simulink model "bike_model_lqrTuning"  (R2018b)
settings: Solver=FixedStepAuto  StartTime=0.0  StopTime=sim_time  FixedStep=Ts_IMU  MaxStep=Ts  RelTol=1e-3
values from neighbouring files (symbols this model uses):
  A = [0      0            1 ... (first row only)    [lqr_design.m]
  B = [0; 1; (a_real*v*sin(lambda_real))/(h_real*b_real)]    [lqr_design.m]
  b_compFilter = 1.095    [configuration.m]    (also in configuration_lqrTuning.m)
  b_real = 1.095    [configuration.m]    (also in configuration_lqrTuning.m)
  g = 9.81    [configuration.m]    (also in configuration_lqrTuning.m)
  IMU_height_real = 0.45    [configuration.m]    (also in configuration_lqrTuning.m)
  initial_states = [deg2rad(2) deg2rad(0) deg2rad(0)]    [configuration.m]    (also in configuration_lqrTuning.m = [deg2rad(0) deg2rad(0) deg2rad(0)])
  input_velocity = 3    [configuration.m]    (also in configuration_lqrTuning.m = 4)
  lambda_compFilter = deg2rad(70)    [configuration.m]    (also in configuration_lqrTuning.m)
  lambda_real = deg2rad(70)    [configuration.m]    (also in configuration_lqrTuning.m)
  lqr_gains = zeros(length(velocity_lqr),3)    [lqr_design.m]
  parameters_compFilter = [g h_compFilter b_compFilter a_compFilter lambda_compFilter c_compFilter]    [configuration.m]    (also in configuration_lqrTuning.m)
  parameters_f_b_real = [m_frame_real m_box_real h_frame_real h_box_real a_frame_real a_box_real c_frame_real c_box_real b_frame_real b_box_real l_frame_real l_box_real]    [configuration.m]    (also in configuration_lqrTuning.m)
  parameters_real = [g h_real b_real a_real lambda_real c_real]    [configuration.m]    (also in configuration_lqrTuning.m)
  plant_model = 1    [configuration.m]    (also in configuration_lqrTuning.m = 2)
  sys_con = ss(A,B,C,D)    [lqr_design.m]
  sys_dis = c2d(sys_con,Ts)    [lqr_design.m]
  Ts = 0.04    [configuration.m]    (also in configuration_lqrTuning.m)
  Ts_IMU = 0.04    [configuration.m]    (also in configuration_lqrTuning.m)
  velocity_lqr = linspace(1.5,10,1000)    [lqr_design.m]
undefined symbols (not defined in the file or in its folder): DiscIntNeverNeededParam, initial_x, initial_y, path_x, path_y
libraries: simulink x4
settings Model: Creator=Boaz Ash  LastModifiedBy=maximef
settings DebuggingCC: UnconnectedInputMsg=none  UnconnectedOutputMsg=none  UnconnectedLineMsg=none  LibraryContextMissingDiagnostic=none
settings SFSimCC: SimUseLocalCustomCode=off
settings RTWCC: RTWUseLocalCustomCode=off

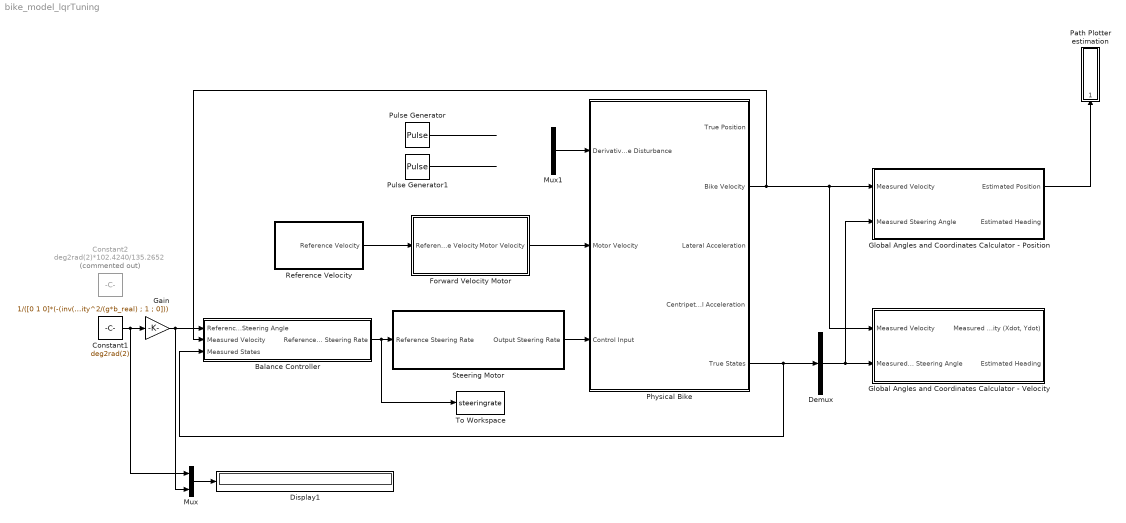
== system bike_model_lqrTuning ==
  Balance Controller : Subsystem  TreatAsAtomicUnit=on  SystemSampleTime=Ts
  Constant1 : Constant  Value=deg2rad(2)
  Constant2 : Constant  Commented=on  Value=deg2rad(2)*102.4240/135.2652
  Demux : Demux  Outputs=3
  Display1 : Display
  Forward Velocity Motor : Subsystem
  Gain : Gain  Gain=1/([0 1 0]*(-(inv(A-B*lqr_gains))*B*lqr_gains*[-input_velocity^2/(g*b_real) ; 1 ; 0]))
  Global Angles and Coordinates Calculator - Position : Subsystem  SystemSampleTime=Ts
  Global Angles and Coordinates Calculator - Velocity : Subsystem  SystemSampleTime=Ts
  Mux : Mux  Inputs=2
  Mux1 : Mux  Inputs=3
  Path Plotter estimation : Subsystem  SystemSampleTime=Ts
  Physical Bike : Subsystem
  Pulse Generator : DiscretePulseGenerator  PulseType=Time based  Amplitude=pi/36  Period=100  PhaseDelay=1
  Pulse Generator1 : DiscretePulseGenerator  PulseType=Time based  Amplitude=-deg2rad(30)  Period=10  PulseWidth=10  PhaseDelay=1
  "Reference Velocity " : Subsystem
  Steering Motor : Subsystem
  To Workspace : ToWorkspace  VariableName=steeringrate  SaveFormat=Timeseries  SampleTime=Ts
  wires:
  Pulse Generator/1 -> ?
  Pulse Generator1/1 -> ?
  Physical Bike/2(Bike Velocity) -> Balance Controller/2(Measured Velocity), Global Angles and Coordinates Calculator - Velocity/1(Measured Velocity), Global Angles and Coordinates Calculator - Position/1(Measured Velocity)
  Forward Velocity Motor/1(Motor Velocity) -> Physical Bike/2(Motor Velocity)
  "Reference Velocity "/1(Reference Velocity) -> Forward Velocity Motor/1(Reference Velocity)
  Steering Motor/1(Output Steering Rate) -> Physical Bike/3(Control Input)
  Physical Bike/5(True States) -> Balance Controller/3(Measured States), Demux/1
  Demux/2 -> Global Angles and Coordinates Calculator - Velocity/2("Measured Steering Angle "), Global Angles and Coordinates Calculator - Position/2(Measured Steering Angle)
  Mux1/1 -> Physical Bike/1(Derivative Disturbance)
  Global Angles and Coordinates Calculator - Position/1(Estimated Position) -> Path Plotter estimation/1(Position)
  Balance Controller/1(Reference Steering Rate) -> To Workspace/1, Steering Motor/1(Reference Steering Rate)
  Constant1/1 -> Mux/1, Gain/1
  Gain/1 -> Mux/2, Balance Controller/1(Reference Steering Angle)
  Mux/1 -> Display1/1

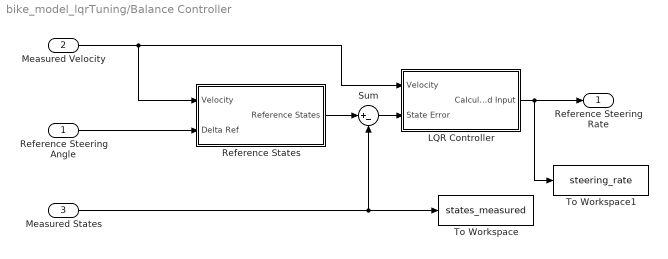
== system bike_model_lqrTuning/Balance Controller ==
  Reference Steering Angle : Inport
  Measured Velocity : Inport  Port=2
  Measured States : Inport  Port=3
  LQR Controller : Subsystem  TreatAsAtomicUnit=on  SystemSampleTime=Ts
  Reference States : Subsystem  SystemSampleTime=Ts
  Sum : Sum  Inputs=|+-
  To Workspace : ToWorkspace  VariableName=states_measured  SaveFormat=Timeseries  SampleTime=-1
  To Workspace1 : ToWorkspace  VariableName=steering_rate  SaveFormat=Timeseries  SampleTime=-1
  Reference Steering Rate : Outport
  wires:
  Reference States/1(Reference States) -> Sum/1
  Sum/1 -> LQR Controller/2(State Error)
  LQR Controller/1(Calculated Input) -> To Workspace1/1, Reference Steering Rate/1
  Reference Steering Angle/1 -> Reference States/2(Delta Ref)
  Measured Velocity/1 -> Reference States/1(Velocity), LQR Controller/1(Velocity)
  Measured States/1 -> To Workspace/1, Sum/2

== system bike_model_lqrTuning/Forward Velocity Motor ==
  note: Add limit for acceleration/deceleration
      | Add min speed of 1.69 m/s (3600 rpm motor speed) limitation
      | Add min speed of 8.20 m/s (18000 rpm motor speed) limitation
      | Add deadband and delay
  Reference Velocity : Inport
  Motor Velocity : Outport
  wires:
  Reference Velocity/1 -> Motor Velocity/1

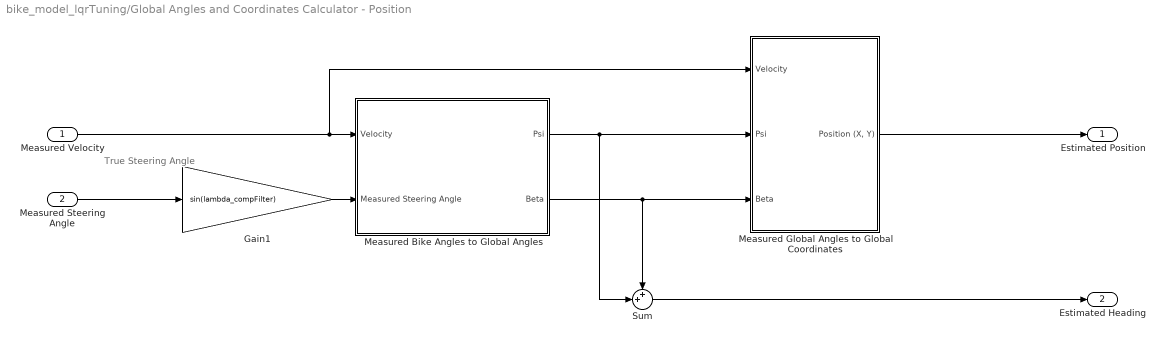
== system bike_model_lqrTuning/Global Angles and Coordinates Calculator - Position ==
  note: True Steering
      | Angle
  Measured Velocity : Inport
  Measured Steering Angle : Inport  Port=2
  Gain1 : Gain  Gain=sin(lambda_compFilter)
  Measured Bike Angles to Global Angles : Subsystem
  Measured Global Angles to Global Coordinates : Subsystem
  Sum : Sum  Inputs=++|
  Estimated Position : Outport
  Estimated Heading : Outport  Port=2
  wires:
  Measured Bike Angles to Global Angles/1(Psi) -> Sum/2, Measured Global Angles to Global Coordinates/2(Psi)
  Gain1/1 -> Measured Bike Angles to Global Angles/2(Measured Steering Angle)
  Sum/1 -> Estimated Heading/1
  Measured Bike Angles to Global Angles/2(Beta) -> Sum/1, Measured Global Angles to Global Coordinates/3(Beta)
  Measured Global Angles to Global Coordinates/1("Position (X, Y)") -> Estimated Position/1
  Measured Velocity/1 -> Measured Global Angles to Global Coordinates/1(Velocity), Measured Bike Angles to Global Angles/1(Velocity)
  Measured Steering Angle/1 -> Gain1/1

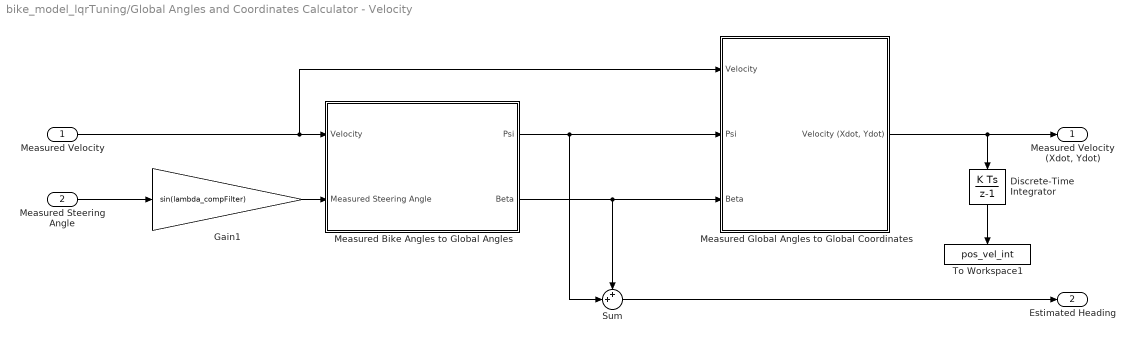
== system bike_model_lqrTuning/Global Angles and Coordinates Calculator - Velocity ==
  Measured Velocity : Inport
  "Measured Steering Angle " : Inport  Port=2
  Discrete-Time Integrator : DiscreteIntegrator  SampleTime=-1  ICPrevOutput=DiscIntNeverNeededParam  ICPrevScaledInput=DiscIntNeverNeededParam
  Gain1 : Gain  Gain=sin(lambda_compFilter)
  Measured Bike Angles to Global Angles : Subsystem
  Measured Global Angles to Global Coordinates : Subsystem
  Sum : Sum  Inputs=++|
  To Workspace1 : ToWorkspace  VariableName=pos_vel_int  SaveFormat=Timeseries  SampleTime=-1
  "Measured Velocity (Xdot, Ydot)" : Outport
  Estimated Heading : Outport  Port=2
  wires:
  "Measured Steering Angle "/1 -> Gain1/1
  Measured Bike Angles to Global Angles/1(Psi) -> Sum/2, Measured Global Angles to Global Coordinates/2(Psi)
  Gain1/1 -> Measured Bike Angles to Global Angles/2(Measured Steering Angle)
  Sum/1 -> Estimated Heading/1
  Measured Bike Angles to Global Angles/2(Beta) -> Measured Global Angles to Global Coordinates/3(Beta), Sum/1
  Measured Velocity/1 -> Measured Bike Angles to Global Angles/1(Velocity), Measured Global Angles to Global Coordinates/1(Velocity)
  Measured Global Angles to Global Coordinates/1("Velocity (Xdot, Ydot)") -> "Measured Velocity (Xdot, Ydot)"/1, Discrete-Time Integrator/1
  Discrete-Time Integrator/1 -> To Workspace1/1

== system bike_model_lqrTuning/Path Plotter estimation ==
  Position : Inport
  Demux : Demux  Outputs=2
  To Workspace : ToWorkspace  VariableName=X_BIKE_estim  SaveFormat=Timeseries  SampleTime=Ts
  To Workspace1 : ToWorkspace  VariableName=Y_BIKE_estim  SaveFormat=Timeseries  SampleTime=Ts
  XY Graph : simulink/Sinks/XY Graph  Commented=on  xmin=min(path_x)-5  xmax=max(path_x)+5  ymin=min(path_y)-5  ymax=max(path_y)+5  st=-1
  wires:
  Demux/1 -> XY Graph/1, To Workspace/1  "X"
  Demux/2 -> XY Graph/2, To Workspace1/1  "Y"
  Position/1 -> Demux/1

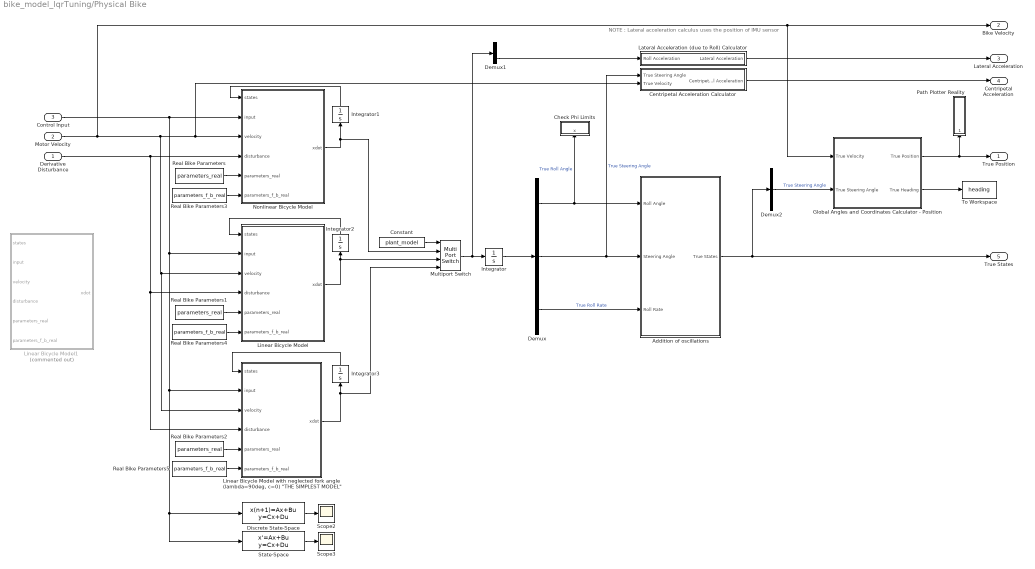
== system bike_model_lqrTuning/Physical Bike ==
  note: NOTE : Lateral acceleration calculus uses the position of IMU sensor
  Derivative Disturbance : Inport
  Motor Velocity : Inport  Port=2
  Control Input : Inport  Port=3
  " Addition of oscillations" : Subsystem  SystemSampleTime=Ts
  Centripetal Acceleration Calculator : Subsystem
  Check Phi Limits : Subsystem  TreatAsAtomicUnit=on  SystemSampleTime=Ts
  Constant : Constant  Value=plant_model
  Demux : Demux  Outputs=3
  Demux1 : Demux  Outputs=3
  Demux2 : Demux  Outputs=3
  Discrete State-Space : DiscreteStateSpace  A=sys_dis.A  B=sys_dis.B  C=eye(3,3)  D=zeros(3,1)  SampleTime=Ts_IMU
  Global Angles and Coordinates Calculator - Position : Subsystem  SystemSampleTime=Ts
  Integrator{,1..3} (4 alike) : Integrator  InitialCondition=initial_states
  Lateral Acceleration (due to Roll) Calculator : Subsystem
  Linear Bicycle Model : MATLAB Function  TreatAsAtomicUnit=on
  "Linear Bicycle Model with neglected fork angle (lambda=90deg, c=0) \"THE SIMPLEST MODEL\"" : MATLAB Function  TreatAsAtomicUnit=on
  Linear Bicycle Model1 : MATLAB Function  Commented=on  TreatAsAtomicUnit=on
  Multiport Switch : MultiPortSwitch
  Nonlinear Bicycle Model : MATLAB Function  TreatAsAtomicUnit=on
  Path Plotter Reality : Subsystem  SystemSampleTime=Ts
  Real Bike Parameters : Constant  Value=parameters_real
  Real Bike Parameters1 : Constant  Value=parameters_real
  Real Bike Parameters2 : Constant  Value=parameters_real
  Real Bike Parameters3 : Constant  Value=parameters_f_b_real
  Real Bike Parameters4 : Constant  Value=parameters_f_b_real
  Real Bike Parameters5 : Constant  Value=parameters_f_b_real
  Scope2 : Scope
  Scope3 : Scope
  State-Space : StateSpace  A=sys_con.A  B=sys_con.B  C=eye(3,3)  D=zeros(3,1)  InitialCondition=0
  To Workspace : ToWorkspace  VariableName=heading  SaveFormat=Timeseries  SampleTime=Ts
  True Position : Outport
  Bike Velocity : Outport  Port=2
  Lateral Acceleration : Outport  Port=3
  Centripetal Acceleration : Outport  Port=4
  True States : Outport  Port=5
  wires:
  Real Bike Parameters5/1 -> "Linear Bicycle Model with neglected fork angle (lambda=90deg, c=0) \"THE SIMPLEST MODEL\""/6(parameters_f_b_real)
  Demux/2 -> Centripetal Acceleration Calculator/1(True Steering Angle), " Addition of oscillations"/2(Steering Angle)  "True Steering Angle"
  Control Input/1 -> Nonlinear Bicycle Model/2(input), State-Space/1, Discrete State-Space/1, "Linear Bicycle Model with neglected fork angle (lambda=90deg, c=0) \"THE SIMPLEST MODEL\""/2(input), Linear Bicycle Model/2(input)
  Integrator1/1 -> Nonlinear Bicycle Model/1(states)
  Real Bike Parameters3/1 -> Nonlinear Bicycle Model/6(parameters_f_b_real)
  Constant/1 -> Multiport Switch/1
  Real Bike Parameters2/1 -> "Linear Bicycle Model with neglected fork angle (lambda=90deg, c=0) \"THE SIMPLEST MODEL\""/5(parameters_real)
  State-Space/1 -> Scope3/1
  Discrete State-Space/1 -> Scope2/1
  Integrator/1 -> Demux/1
  Demux/1 -> Check Phi Limits/1(x), " Addition of oscillations"/1(Roll Angle)  "True Roll Angle"
  Real Bike Parameters1/1 -> Linear Bicycle Model/5(parameters_real)
  Centripetal Acceleration Calculator/1(Centripetal Acceleration) -> Centripetal Acceleration/1
  Nonlinear Bicycle Model/1(xdot) -> Integrator1/1, Multiport Switch/2
  Demux1/3 -> Lateral Acceleration (due to Roll) Calculator/1(Roll Acceleration)
  Linear Bicycle Model/1(xdot) -> Integrator2/1, Multiport Switch/3
  Derivative Disturbance/1 -> Nonlinear Bicycle Model/4(disturbance), "Linear Bicycle Model with neglected fork angle (lambda=90deg, c=0) \"THE SIMPLEST MODEL\""/4(disturbance), Linear Bicycle Model/4(disturbance)
  Real Bike Parameters/1 -> Nonlinear Bicycle Model/5(parameters_real)
  "Linear Bicycle Model with neglected fork angle (lambda=90deg, c=0) \"THE SIMPLEST MODEL\""/1(xdot) -> Integrator3/1, Multiport Switch/4
  Multiport Switch/1 -> Demux1/1, Integrator/1
  Lateral Acceleration (due to Roll) Calculator/1(Lateral Acceleration) -> Lateral Acceleration/1
  Integrator3/1 -> "Linear Bicycle Model with neglected fork angle (lambda=90deg, c=0) \"THE SIMPLEST MODEL\""/1(states)
  Integrator2/1 -> Linear Bicycle Model/1(states)
  Motor Velocity/1 -> Global Angles and Coordinates Calculator - Position/1(True Velocity), Bike Velocity/1, Nonlinear Bicycle Model/3(velocity), Centripetal Acceleration Calculator/2(True Velocity), "Linear Bicycle Model with neglected fork angle (lambda=90deg, c=0) \"THE SIMPLEST MODEL\""/3(velocity), Linear Bicycle Model/3(velocity)
  Real Bike Parameters4/1 -> Linear Bicycle Model/6(parameters_f_b_real)
  Demux/3 -> " Addition of oscillations"/3(Roll Rate)  "True Roll Rate"
  " Addition of oscillations"/1(True States) -> Demux2/1, True States/1
  Demux2/2 -> Global Angles and Coordinates Calculator - Position/2(True Steering Angle)  "True Steering Angle"
  Global Angles and Coordinates Calculator - Position/1(True Position) -> True Position/1, Path Plotter Reality/1(Position)
  Global Angles and Coordinates Calculator - Position/2(True Heading) -> To Workspace/1

== system bike_model_lqrTuning/Reference Velocity  ==
  Constant Velocity : Constant  Value=input_velocity
  Reference Velocity : Outport
  wires:
  Constant Velocity/1 -> Reference Velocity/1

== system bike_model_lqrTuning/Steering Motor ==
  Reference Steering Rate : Inport
  To Workspace : ToWorkspace  VariableName=calculated_input  SaveFormat=Timeseries  SampleTime=Ts
  To Workspace1 : ToWorkspace  VariableName=realised_input  SaveFormat=Timeseries  SampleTime=Ts
  Output Steering Rate : Outport
  wires:
  Reference Steering Rate/1 -> Output Steering Rate/1, To Workspace1/1, To Workspace/1

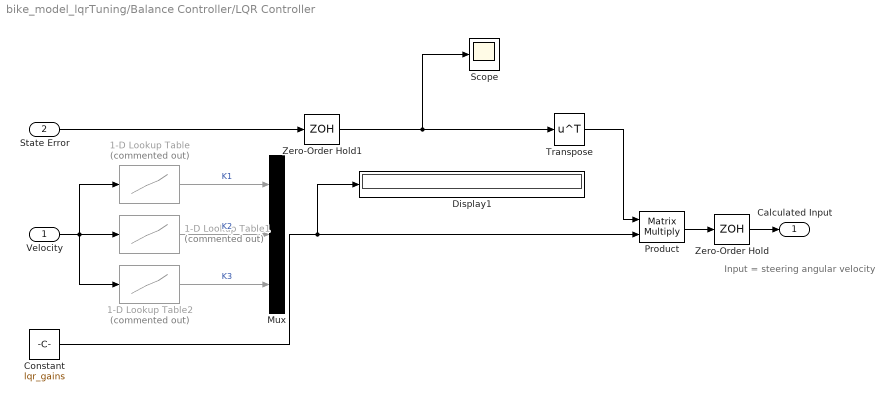
== system bike_model_lqrTuning/Balance Controller/LQR Controller ==
  note: Input = steering angular velocity
  Velocity : Inport
  State Error : Inport  Port=2
  1-D Lookup Table : Lookup_n-D  Commented=on  NumberOfTableDimensions=1  BreakpointsForDimension1=velocity_lqr  BreakpointsForDimension2=velocity_lqr  BreakpointsForDimension3=velocity_lqr  BreakpointsForDimension4=velocity_lqr  Table=lqr_gains(:,1)  InternalRulePriority=Speed  RndMeth=Simplest  InputSameDT=on
  1-D Lookup Table1 : Lookup_n-D  Commented=on  NumberOfTableDimensions=1  BreakpointsForDimension1=velocity_lqr  BreakpointsForDimension2=velocity_lqr  BreakpointsForDimension3=velocity_lqr  BreakpointsForDimension4=velocity_lqr  Table=lqr_gains(:,2)  InternalRulePriority=Speed  RndMeth=Simplest  InputSameDT=on
  1-D Lookup Table2 : Lookup_n-D  Commented=on  NumberOfTableDimensions=1  BreakpointsForDimension1=velocity_lqr  BreakpointsForDimension2=velocity_lqr  BreakpointsForDimension3=velocity_lqr  BreakpointsForDimension4=velocity_lqr  Table=lqr_gains(:,3)  InternalRulePriority=Speed  RndMeth=Simplest  InputSameDT=on
  Constant : Constant  Value=lqr_gains
  Display1 : Display
  Mux : Mux  Inputs=3
  Product : Product  Multiplication=Matrix(*)
  Scope : Scope
  Transpose : Math  Operator=transpose  SaturateOnIntegerOverflow=on
  Zero-Order Hold : ZeroOrderHold  SampleTime=Ts
  Zero-Order Hold1 : ZeroOrderHold  SampleTime=Ts
  Calculated Input : Outport
  wires:
  1-D Lookup Table/1 -> Mux/1  "K1"
  1-D Lookup Table1/1 -> Mux/2  "K2"
  State Error/1 -> Zero-Order Hold1/1
  Product/1 -> Zero-Order Hold/1
  1-D Lookup Table2/1 -> Mux/3  "K3"
  Velocity/1 -> 1-D Lookup Table2/1, 1-D Lookup Table1/1, 1-D Lookup Table/1
  Constant/1 -> Product/2, Display1/1
  Transpose/1 -> Product/1
  Zero-Order Hold/1 -> Calculated Input/1
  Zero-Order Hold1/1 -> Scope/1, Transpose/1

== system bike_model_lqrTuning/Balance Controller/Reference States ==
  Velocity : Inport
  Delta Ref : Inport  Port=2
  Bike Parameters : Constant  Value=parameters_real
  Mux5 : Mux  Inputs=3
  Reference Roll Angle Calculator : MATLAB Function  Commented=on  TreatAsAtomicUnit=on
  Reference Roll Angle Calculator_lin : MATLAB Function  TreatAsAtomicUnit=on
  Reference States : Outport
  wires:
  Bike Parameters/1 -> Reference Roll Angle Calculator_lin/1(parameters_real)
  Delta Ref/1 -> Mux5/2, Reference Roll Angle Calculator_lin/3(delta_ref)
  Reference Roll Angle Calculator_lin/1(phi_ref) -> Mux5/1
  Velocity/1 -> Reference Roll Angle Calculator_lin/2(velocity)
  Mux5/1 -> Reference States/1

== system bike_model_lqrTuning/Global Angles and Coordinates Calculator - Position/Measured Bike Angles to Global Angles ==
  Velocity : Inport
  Measured Steering Angle : Inport  Port=2
  " Bike Parameters Model " : Constant  Value=parameters_compFilter
  Integrator : Integrator
  MATLAB Function : MATLAB Function  TreatAsAtomicUnit=on
  Psi : Outport
  Beta : Outport  Port=2
  wires:
  MATLAB Function/2(beta) -> Beta/1
  MATLAB Function/1(psi_d) -> Integrator/1
  Integrator/1 -> Psi/1
  " Bike Parameters Model "/1 -> MATLAB Function/2(parameters_model)
  Measured Steering Angle/1 -> MATLAB Function/3(delta)
  Velocity/1 -> MATLAB Function/1(v)

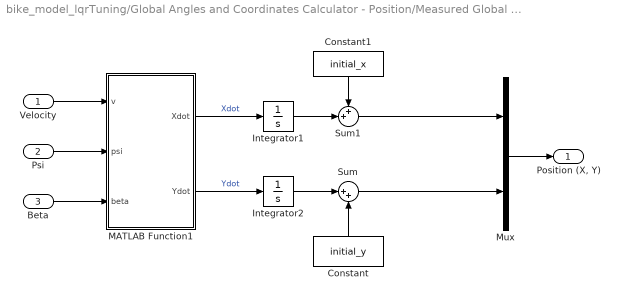
== system bike_model_lqrTuning/Global Angles and Coordinates Calculator - Position/Measured Global Angles to Global Coordinates ==
  Velocity : Inport
  Psi : Inport  Port=2
  Beta : Inport  Port=3
  Constant : Constant  Value=initial_y
  Constant1 : Constant  Value=initial_x
  Integrator1 : Integrator
  Integrator2 : Integrator
  MATLAB Function1 : MATLAB Function  TreatAsAtomicUnit=on
  Mux : Mux  Inputs=2
  Sum : Sum  Inputs=|++
  Sum1 : Sum  Inputs=++|
  "Position (X, Y)" : Outport
  wires:
  MATLAB Function1/2(Ydot) -> Integrator2/1  "Ydot"
  MATLAB Function1/1(Xdot) -> Integrator1/1  "Xdot"
  Psi/1 -> MATLAB Function1/2(psi)
  Beta/1 -> MATLAB Function1/3(beta)
  Velocity/1 -> MATLAB Function1/1(v)
  Integrator2/1 -> Sum/1
  Constant/1 -> Sum/2
  Sum/1 -> Mux/2
  Integrator1/1 -> Sum1/2
  Sum1/1 -> Mux/1
  Constant1/1 -> Sum1/1
  Mux/1 -> "Position (X, Y)"/1

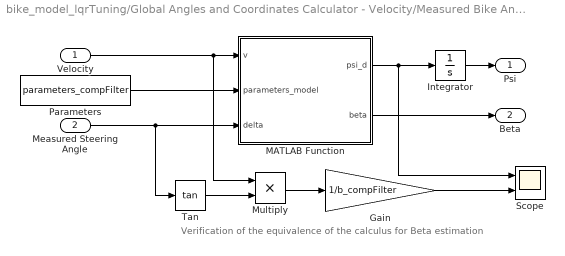
== system bike_model_lqrTuning/Global Angles and Coordinates Calculator - Velocity/Measured Bike Angles to Global Angles ==
  note: Verification of the equivalence of the calculus for Beta estimation
  Velocity : Inport
  Measured Steering Angle : Inport  Port=2
  Gain : Gain  Gain=1/b_compFilter
  Integrator : Integrator
  MATLAB Function : MATLAB Function  TreatAsAtomicUnit=on
  Multiply : Product
  Parameters : Constant  Value=parameters_compFilter
  Scope : Scope  NumInputPorts=2
  Tan : Trigonometry  Operator=tan
  Psi : Outport
  Beta : Outport  Port=2
  wires:
  Integrator/1 -> Psi/1
  MATLAB Function/1(psi_d) -> Scope/1, Integrator/1
  Measured Steering Angle/1 -> Tan/1, MATLAB Function/3(delta)
  Parameters/1 -> MATLAB Function/2(parameters_model)
  Velocity/1 -> Multiply/1, MATLAB Function/1(v)
  MATLAB Function/2(beta) -> Beta/1
  Tan/1 -> Multiply/2
  Multiply/1 -> Gain/1
  Gain/1 -> Scope/2

== system bike_model_lqrTuning/Global Angles and Coordinates Calculator - Velocity/Measured Global Angles to Global Coordinates ==
  Velocity : Inport
  Psi : Inport  Port=2
  Beta : Inport  Port=3
  MATLAB Function1 : MATLAB Function  TreatAsAtomicUnit=on
  Mux1 : Mux  Inputs=2
  "Velocity (Xdot, Ydot)" : Outport
  wires:
  MATLAB Function1/2(Ydot) -> Mux1/2  "Ydot"
  MATLAB Function1/1(Xdot) -> Mux1/1  "Xdot"
  Psi/1 -> MATLAB Function1/2(psi)
  Beta/1 -> MATLAB Function1/3(beta)
  Velocity/1 -> MATLAB Function1/1(v)
  Mux1/1 -> "Velocity (Xdot, Ydot)"/1

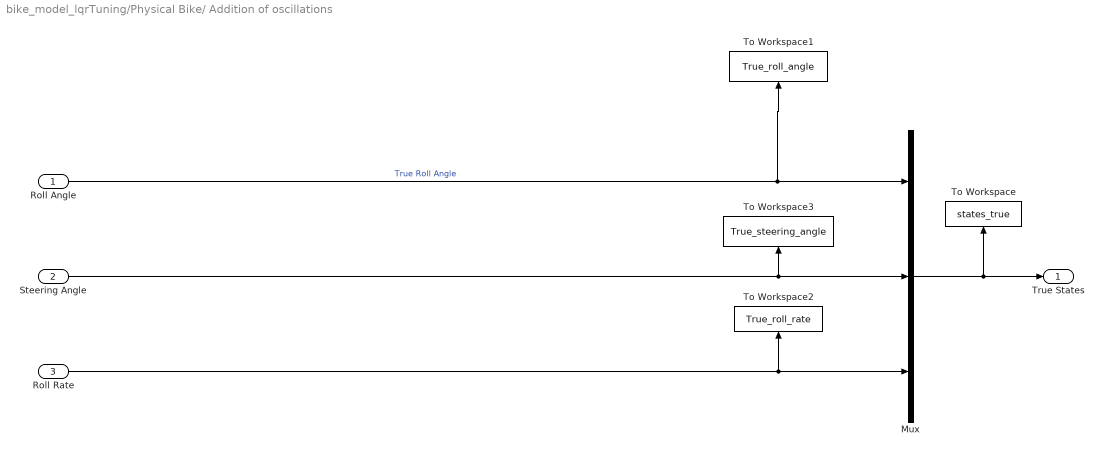
== system bike_model_lqrTuning/Physical Bike/ Addition of oscillations ==
  Roll Angle : Inport
  Steering Angle : Inport  Port=2
  Roll Rate : Inport  Port=3
  Mux : Mux  Inputs=3
  To Workspace : ToWorkspace  VariableName=states_true  SaveFormat=Timeseries  SampleTime=Ts
  To Workspace1 : ToWorkspace  VariableName=True_roll_angle  SaveFormat=Structure  SampleTime=Ts
  To Workspace2 : ToWorkspace  VariableName=True_roll_rate  SaveFormat=Structure  SampleTime=Ts
  To Workspace3 : ToWorkspace  VariableName=True_steering_angle  SaveFormat=Structure  SampleTime=-1
  True States : Outport
  wires:
  Steering Angle/1 -> To Workspace3/1, Mux/2
  Roll Rate/1 -> Mux/3, To Workspace2/1
  Roll Angle/1 -> To Workspace1/1, Mux/1  "True Roll Angle"
  Mux/1 -> True States/1, To Workspace/1

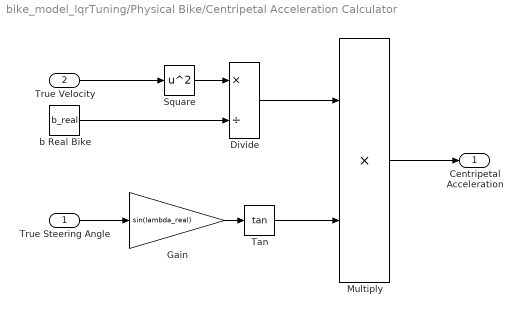
== system bike_model_lqrTuning/Physical Bike/Centripetal Acceleration Calculator ==
  True Steering Angle : Inport
  True Velocity : Inport  Port=2
  Divide : Product  Inputs=*/
  Gain : Gain  Gain=sin(lambda_real)
  Multiply : Product
  Square : Math  Operator=square  SaturateOnIntegerOverflow=on
  Tan : Trigonometry  Operator=tan
  b Real Bike : Constant  Value=b_real
  Centripetal Acceleration : Outport
  wires:
  True Velocity/1 -> Square/1
  Square/1 -> Divide/1
  b Real Bike/1 -> Divide/2
  True Steering Angle/1 -> Gain/1
  Divide/1 -> Multiply/1
  Tan/1 -> Multiply/2
  Multiply/1 -> Centripetal Acceleration/1
  Gain/1 -> Tan/1

== system bike_model_lqrTuning/Physical Bike/Check Phi Limits ==
  x : Inport
  Roll Lower Bound : simulink/Model Verification/Check Static  Lower Bound  Description=min_roll <= u  min=min_roll  min_included=on  enabled=on  stopWhenAssertionFail=on  export=off  icon=graphic
      settings: SourceProductName=Simulink
  Roll Upper Bound : simulink/Model Verification/Check Static  Upper Bound  Description=u <= max_roll  max=max_roll  max_included=on  enabled=on  stopWhenAssertionFail=on  export=off  icon=graphic
      settings: SourceProductName=Simulink  SourceProductBaseCode=SL
  wires:
  x/1 -> Roll Lower Bound/1, Roll Upper Bound/1  "Roll Angle"

== system bike_model_lqrTuning/Physical Bike/Global Angles and Coordinates Calculator - Position ==
  note: True Steering
      | Angle
  True Velocity : Inport
  True Steering Angle : Inport  Port=2
  Gain1 : Gain  Gain=sin(lambda_compFilter)
  Measured Bike Angles to Global Angles : Subsystem
  Measured Global Angles to Global Coordinates : Subsystem
  Sum : Sum  Inputs=++|
  True Position : Outport
  True Heading : Outport  Port=2
  wires:
  Measured Bike Angles to Global Angles/1(Psi) -> Sum/2, Measured Global Angles to Global Coordinates/2(Psi)
  Gain1/1 -> Measured Bike Angles to Global Angles/2(Measured Steering Angle)
  Sum/1 -> True Heading/1
  Measured Bike Angles to Global Angles/2(Beta) -> Sum/1, Measured Global Angles to Global Coordinates/3(Beta)
  Measured Global Angles to Global Coordinates/1("Position (X, Y)") -> True Position/1
  True Velocity/1 -> Measured Global Angles to Global Coordinates/1(Velocity), Measured Bike Angles to Global Angles/1(Velocity)
  True Steering Angle/1 -> Gain1/1

== system bike_model_lqrTuning/Physical Bike/Lateral Acceleration (due to Roll) Calculator ==
  Roll Acceleration : Inport
  Constant3 : Constant  Value=IMU_height_real
  Multiply : Product
  Lateral Acceleration : Outport
  wires:
  Multiply/1 -> Lateral Acceleration/1
  Constant3/1 -> Multiply/1
  Roll Acceleration/1 -> Multiply/2

== system bike_model_lqrTuning/Physical Bike/Path Plotter Reality ==
  Position : Inport
  Demux : Demux  Outputs=2
  To Workspace : ToWorkspace  VariableName=X_BIKE  SaveFormat=Timeseries  SampleTime=Ts
  To Workspace1 : ToWorkspace  VariableName=Y_BIKE  SaveFormat=Timeseries  SampleTime=Ts
  XY Graph : simulink/Sinks/XY Graph  Commented=on  xmin=min(path_x)-5  xmax=max(path_x)+5  ymin=min(path_y)-5  ymax=max(path_y)+5  st=-1
  wires:
  Demux/1 -> XY Graph/1, To Workspace/1  "X"
  Demux/2 -> XY Graph/2, To Workspace1/1  "Y"
  Position/1 -> Demux/1

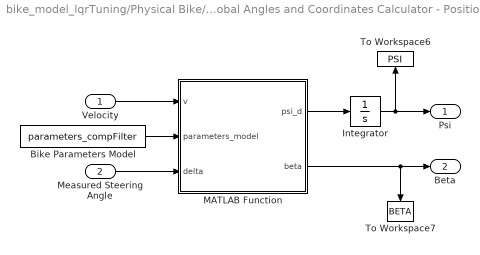
== system bike_model_lqrTuning/Physical Bike/Global Angles and Coordinates Calculator - Position/Measured Bike Angles to Global Angles ==
  Velocity : Inport
  Measured Steering Angle : Inport  Port=2
  " Bike Parameters Model " : Constant  Value=parameters_compFilter
  Integrator : Integrator
  MATLAB Function : MATLAB Function  TreatAsAtomicUnit=on
  To Workspace6 : ToWorkspace  VariableName=PSI  SaveFormat=Timeseries  SampleTime=Ts
  To Workspace7 : ToWorkspace  VariableName=BETA  SaveFormat=Timeseries  SampleTime=Ts
  Psi : Outport
  Beta : Outport  Port=2
  wires:
  MATLAB Function/2(beta) -> Beta/1, To Workspace7/1
  MATLAB Function/1(psi_d) -> Integrator/1
  Integrator/1 -> Psi/1, To Workspace6/1
  " Bike Parameters Model "/1 -> MATLAB Function/2(parameters_model)
  Measured Steering Angle/1 -> MATLAB Function/3(delta)
  Velocity/1 -> MATLAB Function/1(v)

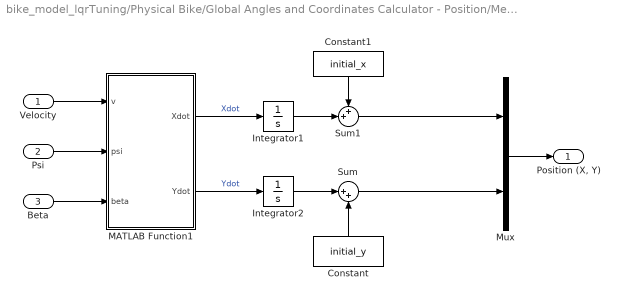
== system bike_model_lqrTuning/Physical Bike/Global Angles and Coordinates Calculator - Position/Measured Global Angles to Global Coordinates ==
  Velocity : Inport
  Psi : Inport  Port=2
  Beta : Inport  Port=3
  Constant : Constant  Value=initial_y
  Constant1 : Constant  Value=initial_x
  Integrator1 : Integrator
  Integrator2 : Integrator
  MATLAB Function1 : MATLAB Function  TreatAsAtomicUnit=on
  Mux : Mux  Inputs=2
  Sum : Sum  Inputs=|++
  Sum1 : Sum  Inputs=++|
  "Position (X, Y)" : Outport
  wires:
  MATLAB Function1/2(Ydot) -> Integrator2/1  "Ydot"
  MATLAB Function1/1(Xdot) -> Integrator1/1  "Xdot"
  Psi/1 -> MATLAB Function1/2(psi)
  Beta/1 -> MATLAB Function1/3(beta)
  Velocity/1 -> MATLAB Function1/1(v)
  Integrator2/1 -> Sum/1
  Constant/1 -> Sum/2
  Sum/1 -> Mux/2
  Integrator1/1 -> Sum1/2
  Sum1/1 -> Mux/1
  Constant1/1 -> Sum1/1
  Mux/1 -> "Position (X, Y)"/1

== matlab function bike_model_lqrTuning/Balance Controller/Reference States/Reference Roll Angle Calculator_lin ==
  data: parameters_real input; velocity input; delta_ref input; phi_ref output
function phi_ref = fcn(parameters_real, velocity, delta_ref)
g = parameters_real(1);
b = parameters_real(3);
v = velocity;

phi_ref = -(v^2 / (g * b) * delta_ref); % tan(theta_ref));

== matlab function bike_model_lqrTuning/Physical Bike/Linear Bicycle Model ==
  data: states input; input input; xdot output; velocity input; disturbance input; parameters_real input; parameters_f_b_real input
function xdot = fcn(states,input,velocity,disturbance,parameters_real,parameters_f_b_real)

delta_d=input;
v=velocity;
d1=disturbance(1);
d2=disturbance(2);
d3=disturbance(3);

% % % 1=frame | 2=box
% % m1=parameters_f_b_real(1);
% % m2=parameters_f_b_real(2);
% % h1=parameters_f_b_real(3);
% % h2=parameters_f_b_real(4);
% % a1=parameters_f_b_real(5);
% % a2=parameters_f_b_real(6);
% % c1=parameters_f_b_real(7);
% % c2=parameters_f_b_real(8);
% % b1=parameters_f_b_real(9);
% % b2=parameters_f_b_real(10);
% % l1=parameters_f_b_real(11);
% % l2=parameters_f_b_real(12);

% 1=frame | 2=box
m1=parameters_real(1);
m2=parameters_real(1);
h1=parameters_real(2);
h2=parameters_real(2);
a1=parameters_real(3);
a2=parameters_real(3);
c1=parameters_real(4);
c2=parameters_real(4);
b1=parameters_real(5);
b2=parameters_real(5);
l1=parameters_real(6);
l2=parameters_real(6);

g=parameters_real(1);
h=parameters_real(2);
b=parameters_real(3);
a=parameters_real(4);
lambda=parameters_real(5);
c=parameters_real(6);

phi=states(1);
delta=states(2);
phi_d=states(3);

A=((m1/12)*((c1^2)+(b1^2)))+(m1*(h1^2))+((m2/12)*((c2^2)+(b2^2)))+(m2*(h2^2));
B=((m1/12)*((l1^2)+(b1^2)))-(m1*a1*h1)+((m2/12)*((c2^2)+(b2^2)))+(m2*a2*h2);
D=(((m1*h1)+(m2*h2))*(v^2))-(c*g*((m1*a1)-(m2*a2)));

xdot1=phi_d+d1;
xdot2=delta_d+d2;
% xdot3=((((m1*h1)+(m2*h2))*g)/A)*phi+((D*sin(lambda))/(b*A))*delta+d3+((B*v*sin(lambda))/(b*A))*delta_d;
xdot3=(g/h)*phi+(sin(lambda)*(h*v^2-g*a*c)/(h^2*b))*delta+d3+((a*v*sin(lambda))/(h*b))*delta_d;

xdot=[xdot1 xdot2 xdot3];

== matlab function bike_model_lqrTuning/Global Angles and Coordinates Calculator - Position/Measured Bike Angles to Global Angles/MATLAB Function ==
  data: v input; parameters_model input; delta input; psi_d output; beta output
function [psi_d, beta]  = fcn(v, parameters_model, delta)

b = parameters_model(3);
a = parameters_model(4);

beta = atan((a / (b)) * tan(delta));
psi_d = (v / a) * sin(beta);

== matlab function bike_model_lqrTuning/Physical Bike/Linear Bicycle Model1 ==
  data: states input; input input; xdot output; velocity input; disturbance input; parameters_real input; parameters_f_b_real input
function xdot = fcn(states,input,velocity,disturbance,parameters_real,parameters_f_b_real)

delta_d=input;
v=velocity;
d1=disturbance(1);
d2=disturbance(2);
d3=disturbance(3);

% 1=frame | 2=box
m1=parameters_f_b_real(1);
m2=parameters_f_b_real(2);
h1=parameters_f_b_real(3);
h2=parameters_f_b_real(4);
a1=parameters_f_b_real(5);
a2=parameters_f_b_real(6);
c1=parameters_f_b_real(7);
c2=parameters_f_b_real(8);
b1=parameters_f_b_real(9);
b2=parameters_f_b_real(10);
l1=parameters_f_b_real(11);
l2=parameters_f_b_real(12);

g=parameters_real(1);
%h=parameters_real(2);
b=parameters_real(3);
%a=parameters_real(4);
lambda=parameters_real(5);
c=parameters_real(6);

phi=states(1);
delta=states(2);
phi_d=states(3);

A=((m1/12)*((c1^2)+(b1^2)))+(m1*(h1^2))+((m2/12)*((c2^2)+(b2^2)))+(m2*(h2^2));
B=((m1/12)*((l1^2)+(b1^2)))-(m1*a1*h1)+((m2/12)*((c2^2)+(b2^2)))+(m2*a2*h2);
D=(((m1*h1)+(m2*h2))*(v^2))-(c*g*((m1*a1)-(m2*a2)));

xdot1=phi_d+d1;
xdot2=delta_d+d2;
xdot3=((((m1*h1)+(m2*h2))*g)/A)*phi+((D*sin(lambda))/(b*A))*delta+d3+((B*v*sin(lambda))/(b*A))*delta_d;

xdot=[xdot1 xdot2 xdot3];

== matlab function bike_model_lqrTuning/Global Angles and Coordinates Calculator - Position/Measured Global Angles to Global Coordinates/MATLAB Function1 ==
  data: v input; psi input; Xdot output; beta input; Ydot output
function [Xdot, Ydot]  = fcn(v, psi, beta)

Xdot = v * cos(psi + beta);
Ydot = v * sin(psi + beta);

== matlab function bike_model_lqrTuning/Balance Controller/Reference States/Reference Roll Angle Calculator ==
  data: parameters_real input; velocity input; delta_ref input; phi_ref output
function phi_ref = fcn(parameters_real, velocity, delta_ref)
g = parameters_real(1);
b = parameters_real(3);
v = velocity;

phi_ref = -atan(v^2 / (g * b) * delta_ref); % tan(theta_ref));

== matlab function bike_model_lqrTuning/Physical Bike/Global Angles and Coordinates Calculator - Position/Measured Bike Angles to Global Angles/MATLAB Function ==
  data: v input; parameters_model input; delta input; psi_d output; beta output
function [psi_d, beta]  = fcn(v, parameters_model, delta)

b = parameters_model(3);
a = parameters_model(4);

beta = atan((a / (b)) * tan(delta));
psi_d = (v / a) * sin(beta);

== matlab function bike_model_lqrTuning/Physical Bike/Nonlinear Bicycle Model ==
  data: states input; input input; xdot output; velocity input; disturbance input; parameters_real input; parameters_f_b_real input
function xdot = fcn(states,input,velocity,disturbance,parameters_real,parameters_f_b_real)

delta_d=input;
v=velocity;
d1=disturbance(1);
d2=disturbance(2);
d3=disturbance(3);

% 1=frame | 2=box
m1=parameters_f_b_real(1);
m2=parameters_f_b_real(2);
h1=parameters_f_b_real(3);
h2=parameters_f_b_real(4);
a1=parameters_f_b_real(5);
a2=parameters_f_b_real(6);
c1=parameters_f_b_real(7);
c2=parameters_f_b_real(8);
b1=parameters_f_b_real(9);
b2=parameters_f_b_real(10);
l1=parameters_f_b_real(11);
l2=parameters_f_b_real(12);


g=parameters_real(1);
%h=parameters_real(2);
b=parameters_real(3);
%a=parameters_real(4);
lambda=parameters_real(5);
c=parameters_real(6);

A=((m1/12)*((c1^2)+(b1^2)))+(m1*(h1^2))+((m2/12)*((c2^2)+(b2^2)))+(m2*(h2^2));
B=(m1*a1*h1)-(m2*a2*h2);
D=(((m1*h1)+(m2*h2))*(v^2))-(c*g*((m1*a1)-(m2*a2)));

phi=states(1);
delta=states(2);
phi_d=states(3);


% Biaised mass from box mass measurement
% m = 9.3;
% d = 0.03;
% T = m*d*g*cos(phi)/A;
% % T = 0;

% Biaised mass from bike equilibrium measurement
m = 9.3;
d = 0.07;
T = m*d*g*cos(phi)/A;
T = 0;

xdot1=phi_d+d1;
xdot2=delta_d+d2;
xdot3=((((m1*h1)+(m2*h2))*g)/A)*tan(phi) - T +((D*sin(lambda))/(b*A))*tan(delta)+d3+((B*v*sin(lambda))/(b*A))*tan(delta_d);

xdot=[xdot1 xdot2 xdot3];

== matlab function bike_model_lqrTuning/Physical Bike/Linear Bicycle Model with neglected fork angle (lambda=90deg, c=0) "THE SIMPLEST MODEL" ==
  data: states input; input input; xdot output; velocity input; disturbance input; parameters_real input; parameters_f_b_real input
function xdot = fcn(states,input,velocity,disturbance,parameters_real,parameters_f_b_real)

delta_d=input;
v=velocity;
d1=disturbance(1);
d2=disturbance(2);
d3=disturbance(3);

% 1=frame | 2=box
m1=parameters_f_b_real(1);
m2=parameters_f_b_real(2);
h1=parameters_f_b_real(3);
h2=parameters_f_b_real(4);
a1=parameters_f_b_real(5);
a2=parameters_f_b_real(6);
c1=parameters_f_b_real(7);
c2=parameters_f_b_real(8);
b1=parameters_f_b_real(9);
b2=parameters_f_b_real(10);
l1=parameters_f_b_real(11);
l2=parameters_f_b_real(12);

g=parameters_real(1);
%h=parameters_real(2);
b=parameters_real(3);
%a=parameters_real(4);
lambda=parameters_real(5);
c=parameters_real(6);

A=((m1/12)*((c1^2)+(b1^2)))+(m1*(h1^2))+((m2/12)*((c2^2)+(b2^2)))+(m2*(h2^2));
B=((m1/12)*((l1^2)+(b1^2)))-(m1*a1*h1)+((m2/12)*((c2^2)+(b2^2)))+(m2*a2*h2);
D=(((m1*h1)+(m2*h2))*(v^2))-(c*g*((m1*a1)-(m2*a2)));

phi=states(1);
delta=states(2);
phi_d=states(3);

xdot1=phi_d+d1;
xdot2=delta_d+d2;
xdot3=((((m1*h1)+(m2*h2))*g)/A)*phi+((D*sin(lambda))/(b*A))*delta+d3+((B*v*sin(lambda))/(b*A))*delta_d;

xdot=[xdot1 xdot2 xdot3];

== matlab function bike_model_lqrTuning/Global Angles and Coordinates Calculator - Velocity/Measured Bike Angles to Global Angles/MATLAB Function ==
  data: v input; parameters_model input; delta input; psi_d output; beta output
function [psi_d, beta]  = fcn(v, parameters_model, delta)

b = parameters_model(3);
a = parameters_model(4);

beta = atan((a / (b)) * tan(delta));
psi_d = (v / a) * sin(beta);

== matlab function bike_model_lqrTuning/Global Angles and Coordinates Calculator - Velocity/Measured Global Angles to Global Coordinates/MATLAB Function1 ==
  data: v input; psi input; Xdot output; beta input; Ydot output
function [Xdot, Ydot]  = fcn(v, psi, beta)

Xdot = v * cos(psi + beta);
Ydot = v * sin(psi + beta);

== matlab function bike_model_lqrTuning/Physical Bike/Global Angles and Coordinates Calculator - Position/Measured Global Angles to Global Coordinates/MATLAB Function1 ==
  data: v input; psi input; Xdot output; beta input; Ydot output
function [Xdot, Ydot]  = fcn(v, psi, beta)

Xdot = v * cos(psi + beta);
Ydot = v * sin(psi + beta);
